simulink model "egorov"  (R2024a)
settings: Solver=VariableStepAuto  StartTime=0.0  StopTime=1000  RelTol=1e-3
settings Model: Creator=Lore2  LastModifiedBy=Lore2

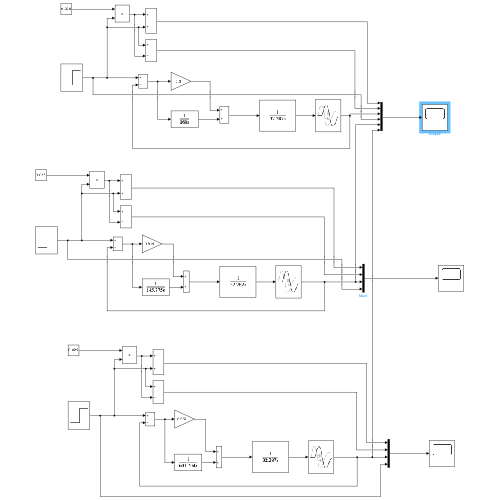
[thumbnail: Simulink's stored preview of the top-level diagram]
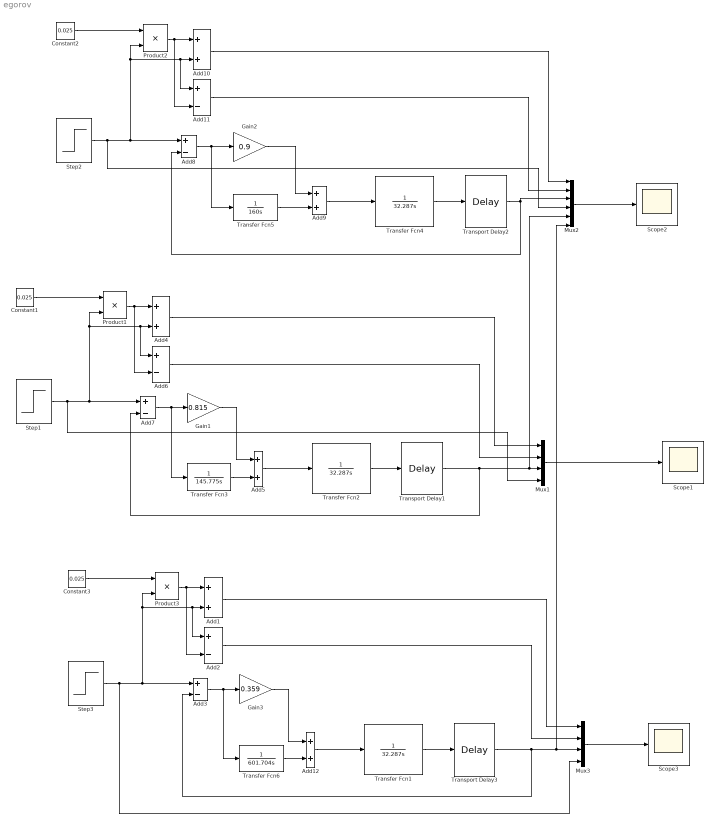
== system egorov ==
  Add{1,4..5,9..10,12} (6 alike) : Sum
  Add{2..3,6..8,11} (6 alike) : Sum  Inputs=+-
  Constant1 : Constant  Value=0.025
  Constant2 : Constant  Value=0.025
  Constant3 : Constant  Value=0.025
  Gain1 : Gain  Gain=0.815
  Gain2 : Gain  Gain=0.9
  Gain3 : Gain  Gain=0.359
  Mux1 : Mux
  Mux2 : Mux  Inputs=6
  Mux3 : Mux
  Product1 : Product
  Product2 : Product
  Product3 : Product
  Scope1 : Scope
  Scope2 : Scope
  Scope3 : Scope
  Step1 : Step  SampleTime=0
  Step2 : Step  SampleTime=0
  Step3 : Step  SampleTime=0
  Transfer Fcn1 : TransferFcn  Denominator=[32.287 0]
  Transfer Fcn2 : TransferFcn  Denominator=[32.287 0]
  Transfer Fcn3 : TransferFcn  Denominator=[145.775 0]
  Transfer Fcn4 : TransferFcn  Denominator=[32.287 0]
  Transfer Fcn5 : TransferFcn  Denominator=[160 0]
  Transfer Fcn6 : TransferFcn  Denominator=[601.704 0]
  Transport Delay1 : TransportDelay  DelayTime=36.002
  Transport Delay2 : TransportDelay  DelayTime=36.002
  Transport Delay3 : TransportDelay  DelayTime=36.002
  wires:
  Add10/1 -> Mux2/1
  Mux2/1 -> Scope2/1
  Product2/1 -> Add11/2, Add10/1
  Gain2/1 -> Add9/1
  Add11/1 -> Mux2/2
  Transport Delay2/1 -> Add8/2, Mux2/3
  Constant2/1 -> Product2/1
  Add9/1 -> Transfer Fcn4/1
  Transfer Fcn5/1 -> Add9/2
  Transfer Fcn4/1 -> Transport Delay2/1
  Step2/1 -> Mux2/4, Add11/1, Add10/2, Product2/2, Add8/1
  Add8/1 -> Transfer Fcn5/1, Gain2/1
  Mux3/1 -> Scope3/1
  Add1/1 -> Mux3/1
  Transfer Fcn6/1 -> Add12/2
  Step3/1 -> Mux3/4, Add2/1, Add1/2, Product3/2, Add3/1
  Transfer Fcn1/1 -> Transport Delay3/1
  Add12/1 -> Transfer Fcn1/1
  Transport Delay3/1 -> Add3/2, Mux2/6, Mux3/3
  Add3/1 -> Transfer Fcn6/1, Gain3/1
  Constant3/1 -> Product3/1
  Product3/1 -> Add2/2, Add1/1
  Gain3/1 -> Add12/1
  Add2/1 -> Mux3/2
  Gain1/1 -> Add5/1
  Add6/1 -> Mux1/2
  Transfer Fcn3/1 -> Add5/2
  Product1/1 -> Add6/2, Add4/1
  Transport Delay1/1 -> Add7/2, Mux2/5, Mux1/3
  Add7/1 -> Transfer Fcn3/1, Gain1/1
  Constant1/1 -> Product1/1
  Transfer Fcn2/1 -> Transport Delay1/1
  Step1/1 -> Mux1/4, Add6/1, Add4/2, Product1/2, Add7/1
  Add5/1 -> Transfer Fcn2/1
  Add4/1 -> Mux1/1
  Mux1/1 -> Scope1/1
